simulink model "thermostat"  (Simulink 4.00)
settings: Solver=ode45  StartTime=0.0  StopTime=10.0  RelTol=1e-3
settings Model: LastModifiedBy=hespanha  BlockReductionOpt=off

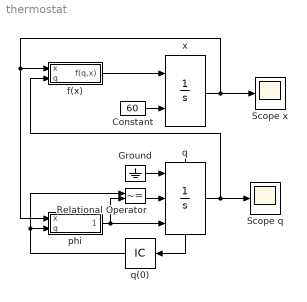
== system thermostat ==
  Constant : Constant  Value=60
  Ground : Ground
  Relational Operator : RelationalOperator  Operator=~=
  Scope q : Scope
      settings: TimeRange=10  YMin=0  YMax=3  SaveToWorkspace=off  LimitDataPoints=on  MaxDataPoints=5000
  Scope x : Scope
      settings: TimeRange=10  YMin=60  YMax=80  SaveToWorkspace=off  SaveName=ScopeData  LimitDataPoints=on  MaxDataPoints=5000
  f(x) : Subsystem  Description=f(x)
      settings: RTWFcnNameOpts=Auto  RTWFileNameOpts=Auto
  phi : Subsystem  Description=f(x)
      settings: RTWFcnNameOpts=Auto  RTWFileNameOpts=Auto
  q : Integrator  ExternalReset=rising  InitialConditionSource=external  InitialCondition=0  LimitOutput=off  UpperSaturationLimit=inf  LowerSaturationLimit=-inf  ShowSaturationPort=off  ShowStatePort=on  AbsoluteTolerance=auto
  q(0) : InitialCondition  Orientation=left  Value=1
  x : Integrator  ExternalReset=none  InitialConditionSource=external  InitialCondition=0  LimitOutput=off  UpperSaturationLimit=inf  LowerSaturationLimit=-inf  ShowSaturationPort=off  ShowStatePort=off  AbsoluteTolerance=auto
  wires:
  Constant/1 -> x/2
  f(x)/1(f(q,x)) -> x/1
  x/1 -> Scope x/1, phi/1(x), f(x)/1(x)
  q/1 -> Scope q/1, f(x)/2(q)
  Ground/1 -> q/1
  Relational Operator/1 -> q/2
  phi/1(phi(q,x)) -> q/3, Relational Operator/2
  q(0)/1 -> phi/2(q), Relational Operator/1
  q/State -> q(0)/1

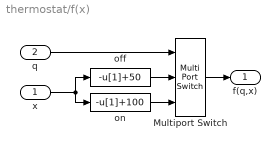
== system thermostat/f(x) ==
  x : Inport  Port=1
  q : Inport  Port=2
  Multiport Switch : MultiPortSwitch  Inputs=2
  off : Fcn  Expr=-u[1]+50
  on : Fcn  Expr=-u[1]+100
  f(q,x) : Outport  Port=1
  wires:
  Multiport Switch/1 -> f(q,x)/1
  off/1 -> Multiport Switch/2
  on/1 -> Multiport Switch/3
  x/1 -> off/1, on/1
  q/1 -> Multiport Switch/1

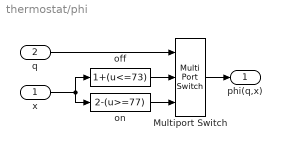
== system thermostat/phi ==
  x : Inport  Port=1
  q : Inport  Port=2
  Multiport Switch : MultiPortSwitch  Inputs=2
  off : Fcn  Expr=1+(u<=73)
  on : Fcn  Expr=2-(u>=77)
  phi(q,x) : Outport  Port=1
  wires:
  x/1 -> on/1, off/1
  on/1 -> Multiport Switch/3
  off/1 -> Multiport Switch/2
  Multiport Switch/1 -> phi(q,x)/1
  q/1 -> Multiport Switch/1
